simulink model "Even_Software_rezontor_original"  (R2019a)
settings: Solver=VariableStepAuto  StartTime=0.0  StopTime=20  FixedStep=0.000001  RelTol=1e-3
libraries: simulink x1
settings Model: NumberOfSteps=16  Creator=vardhah  LastModifiedBy=vardhah
settings DataIOCC: ReturnWorkspaceOutputs=off
settings DebuggingCC: UnderSpecifiedDimensionMsg=warning  ArithmeticOperatorsInVariantConditions=warning

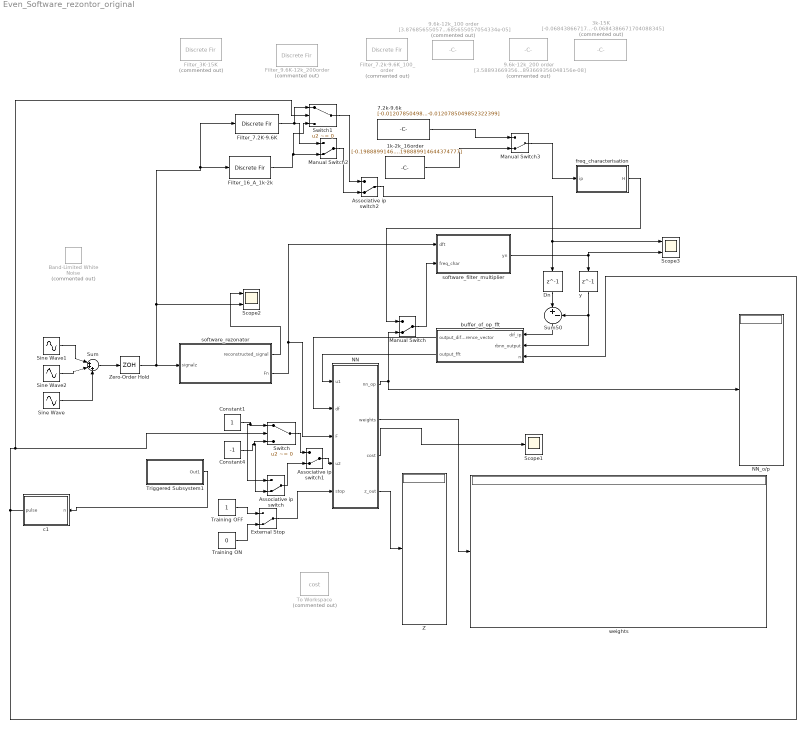
== system Even_Software_rezontor_original ==
  1k-2k_16order : Constant  Value=[-0.198889914644374777 0.0882189428518377339 0.0736891495871065116 0.0638368801789635787 0.0566372642221577294 0.0523172683654103132 0.0494565343907736044 0.048157521822162791 0.048157521822162791 0.0494565343907736044 0.0523172683654103132 0.0566372642221577294 0.0638368801789635787 0.0736891495871065116 0.0882189428518377339 -0.198889914644374777]  VectorParams1D=off
  3k-15K : Constant  Commented=on  Value=[-0.0684386671704088345 -0.0216035519389094557 -0.0869907772510868094 -0.0695372998678755599 0.0160068430386171648 -0.171506412844009415 -0.104404398490726372 0.48413102780480427 0.48413102780480427 -0.104404398490726372 -0.171506412844009415 0.0160068430386171648 -0.0695372998678755599 -0.0869907772510868094 -0.0216035519389094557 -0.0684386671704088345]  VectorParams1D=off
  "7.2k-9.6k " : Constant  Value=[-0.0120785049852322399 -0.0942455273574688279 0.0101245004695954266 0.125460404555770566 0.034165372769331126 -0.1614987160724079 -0.0984930555982914957 0.150982315564688691 0.150982315564688691 -0.0984930555982914957 -0.1614987160724079 0.034165372769331126 0.125460404555770566 0.0101245004695954266 -0.0942455273574688279 -0.0120785049852322399]  VectorParams1D=off
  9.6k-12k_100 order : Constant  Commented=on  Value=[3.87685655057054334e-05 0.000108803053226908729 -8.26167990877867136e-05 -0.000293336203733274498 2.6285942662608911e-05 0.000470643257144739719 0.000128704829547001234 -0.000409932472117148169 -0.000168878837800233775 5.29388077798551043e-06 -0.000285438581748162664 0.000476496961661710902 0.00138356120682394616 -0.000476433595901257331 -0.00260989841330203781 -0.000263832520003181659 0.00288776740876196033 0.00103696232298899297 -0.00148535664212565491 -0.00029781571721707251 -0.000910294888597508478 -0.00301220003423313329 0.00221471961553778218 0.00782175074594450466 -0.000709211369068674449 -0.0107696105008747954 -0.00258145844866515843 0.00855726436285330835 0.00338081517511367325 -0.00144715698429817813 0.00287506321799563301 -0.00544178445149644165 -0.016125692798747971 0.00552050119563736973 0.0291833518348223603 0.00265487109805798843 -0.0313375380418604021 -0.0109425432817974923 0.0170337904278449956 0.00463136074451602191 0.00673385154025073988 0.0271658069884841494 -0.0215094126752095813 -0.080672987166974186 0.00848125715451410883 0.135328268501058141 0.0372155688614851238 -0.164113227506699488 -0.099857601639362345 0.150463696417151488 0.150463696417151488 -0.099857601639362345 -0.164113227506699488 0.0372155688614851238 0.135328268501058141 0.00848125715451410883 -0.080672987166974186 -0.0215094126752095813 0.0271658069884841494 0.00673385154025073988 0.00463136074451602191 0.0170337904278449956 -0.0109425432817974923 -0.0313375380418604021 0.00265487109805798843 0.0291833518348223603 0.00552050119563736973 -0.016125692798747971 -0.00544178445149644165 0.00287506321799563301 -0.00144715698429817813 0.00338081517511367325 0.00855726436285330835 -0.00258145844866515843 -0.0107696105008747954 -0.000709211369068674449 0.00782175074594450466 0.00221471961553778218 -0.00301220003423313329 -0.000910294888597508478 -0.00029781571721707251 -0.00148535664212565491 0.00103696232298899297 0.00288776740876196033 -0.000263832520003181659 -0.00260989841330203781 -0.000476433595901257331 0.00138356120682394616 0.000476496961661710902 -0.000285438581748162664 5.29388077798551043e-06 -0.000168878837800233775 -0.000409932472117148169 0.000128704829547001234 0.000470643257144739719 2.6285942662608911e-05 -0.000293336203733274498 -8.26167990877867136e-05 0.000108803053226908729 3.87685655057054334e-05]  VectorParams1D=off
  9.6k-12k_200 order : Constant  Commented=on  Value=[3.58893669356048156e-08 -3.82818873463390521e-08 -2.0321720028023873e-07 4.90359188072874186e-08 5.60695246712035587e-07 1.09660540028249228e-07 -9.02554244437910404e-07 -4.11425973326973434e-07 7.02261176603049468e-07 1.84471216608655933e-07 3.26725285155721724e-07 1.85122942566739851e-06 -1.30883758906231066e-06 -6.26130099657902526e-06 3.05461039932901012e-07 1.09009807667638867e-05 3.23497432520277999e-06 -1.08958455239369133e-05 -4.97738604970975483e-06 2.96863479339988865e-06 -4.0832027868080837e-06 8.18297554751245384e-06 2.96530358064679952e-05 -9.55109847507026519e-06 -6.23922165547140565e-05 -7.71216677200245448e-06 7.59750359409520817e-05 2.93209615001356784e-05 -4.65187720652641962e-05 -1.41370609590419019e-05 -1.56985235131491563e-05 -7.53719240448361523e-05 5.59153495137252289e-05 0.000221327384655395267 -1.66050969068338295e-05 -0.000328656395451828759 -8.51260959631819787e-05 0.000282645117406031716 0.000119666235755805559 -6.72511324233616883e-05 7.71213722411986897e-05 -0.000163098688300092245 -0.000529184616157781082 0.000174782969900715956 0.000998932721197958676 0.000103789032707165716 -0.00109406787912954759 -0.000393069844497760581 0.000605548903230077127 0.00017901057135702881 0.000188671213168486616 0.0008317537932211581 -0.000616428076574026661 -0.00225801358273229787 0.000189644939633113819 0.00309786671618311488 0.000749066198738662951 -0.00246959577998202753 -0.000999305917144800888 0.000543345759446133242 -0.000591058888909330575 0.00125474640273121702 0.00385350017895572799 -0.0012819719093164299 -0.00685815514325687284 -0.000643891365732486565 0.00710257598433050412 0.00245016739238454462 -0.00372825461824609263 -0.00107354982596571057 -0.00112558364252808812 -0.00473944354418633605 0.00351472715485449472 0.0123820578712038748 -0.0011101460878915094 -0.0164148510072775998 -0.00382732465676402251 0.0127139357915301426 0.00503981617377440537 -0.00272012803122949386 0.00293385456875478335 -0.00629326791759583608 -0.0189964846306969505 0.00647240842885716226 0.0339172426787937645 0.00302977722420997957 -0.0357411919442247455 -0.0123754194694439944 0.0194465496197908511 0.00571238915438039823 0.00633940801538525594 0.0275121602229752085 -0.0219528139243238031 -0.0822938722183100269 0.00864574898877375209 0.1372509242650502 0.0376134106872798024 -0.165584050427181245 -0.100574100965544921 0.151437569678198519 0.151437569678198519 -0.100574100965544921 -0.165584050427181245 0.0376134106872798024 0.1372509242650502 0.00864574898877375209 -0.0822938722183100269 -0.0219528139243238031 0.0275121602229752085 0.00633940801538525594 0.00571238915438039823 0.0194465496197908511 -0.0123754194694439944 -0.0357411919442247455 0.00302977722420997957 0.0339172426787937645 0.00647240842885716226 -0.0189964846306969505 -0.00629326791759583608 0.00293385456875478335 -0.00272012803122949386 0.00503981617377440537 0.0127139357915301426 -0.00382732465676402251 -0.0164148510072775998 -0.0011101460878915094 0.0123820578712038748 0.00351472715485449472 -0.00473944354418633605 -0.00112558364252808812 -0.00107354982596571057 -0.00372825461824609263 0.00245016739238454462 0.00710257598433050412 -0.000643891365732486565 -0.00685815514325687284 -0.0012819719093164299 0.00385350017895572799 0.00125474640273121702 -0.000591058888909330575 0.000543345759446133242 -0.000999305917144800888 -0.00246959577998202753 0.000749066198738662951 0.00309786671618311488 0.000189644939633113819 -0.00225801358273229787 -0.000616428076574026661 0.0008317537932211581 0.000188671213168486616 0.00017901057135702881 0.000605548903230077127 -0.000393069844497760581 -0.00109406787912954759 0.000103789032707165716 0.000998932721197958676 0.000174782969900715956 -0.000529184616157781082 -0.000163098688300092245 7.71213722411986897e-05 -6.72511324233616883e-05 0.000119666235755805559 0.000282645117406031716 -8.51260959631819787e-05 -0.000328656395451828759 -1.66050969068338295e-05 0.000221327384655395267 5.59153495137252289e-05 -7.53719240448361523e-05 ...(+757 chars)]  VectorParams1D=off
  Associative ip switch : ManualSwitch  CurrentSetting=0
  Associative ip switch1 : ManualSwitch  CurrentSetting=0
  Associative ip switch2 : ManualSwitch  CurrentSetting=0
  Band-Limited White Noise : simulink/Sources/Band-Limited White Noise  Commented=on  Cov=[2]  Ts=0.000001  seed=[23341]
  Constant1 : Constant
  Constant4 : Constant  Value=-1
  Dn : Delay  DelayLength=1  InitialCondition=0
  External Stop : ManualSwitch  CurrentSetting=0
  Filter_16_A_1k-2k : DiscreteFir  Tag=BlockMethodSubSystem  Coefficients=[-0.198889914644374777 0.0882189428518377339 0.0736891495871065116 0.0638368801789635787 0.0566372642221577294 0.0523172683654103132 0.0494565343907736044 0.048157521822162791 0.048157521822162791 0.0494565343907736044 0.0523172683654103132 0.0566372642221577294 0.0638368801789635787 0.0736891495871065116 0.0882189428518377339 -0.198889914644374777]  InputProcessing=Columns as channels (frame based)
  Filter_3K-15K : DiscreteFir  Tag=BlockMethodSubSystem  Commented=on  Coefficients=[-0.0684386671704088345 -0.0216035519389094557 -0.0869907772510868094 -0.0695372998678755599 0.0160068430386171648 -0.171506412844009415 -0.104404398490726372 0.48413102780480427 0.48413102780480427 -0.104404398490726372 -0.171506412844009415 0.0160068430386171648 -0.0695372998678755599 -0.0869907772510868094 -0.0216035519389094557 -0.0684386671704088345]  InputProcessing=Columns as channels (frame based)
  "Filter_7.2K-9.6K " : DiscreteFir  Tag=BlockMethodSubSystem  Coefficients=[-0.0120785049852322399 -0.0942455273574688279 0.0101245004695954266 0.125460404555770566 0.034165372769331126 -0.1614987160724079 -0.0984930555982914957 0.150982315564688691 0.150982315564688691 -0.0984930555982914957 -0.1614987160724079 0.034165372769331126 0.125460404555770566 0.0101245004695954266 -0.0942455273574688279 -0.0120785049852322399]  InputProcessing=Columns as channels (frame based)
  Filter_7.2k-9.6K_100_order : DiscreteFir  Tag=BlockMethodSubSystem  Commented=on  Coefficients=[3.87685655057054334e-05 0.000108803053226908729 -8.26167990877867136e-05 -0.000293336203733274498 2.6285942662608911e-05 0.000470643257144739719 0.000128704829547001234 -0.000409932472117148169 -0.000168878837800233775 5.29388077798551043e-06 -0.000285438581748162664 0.000476496961661710902 0.00138356120682394616 -0.000476433595901257331 -0.00260989841330203781 -0.000263832520003181659 0.00288776740876196033 0.00103696232298899297 -0.00148535664212565491 -0.00029781571721707251 -0.000910294888597508478 -0.00301220003423313329 0.00221471961553778218 0.00782175074594450466 -0.000709211369068674449 -0.0107696105008747954 -0.00258145844866515843 0.00855726436285330835 0.00338081517511367325 -0.00144715698429817813 0.00287506321799563301 -0.00544178445149644165 -0.016125692798747971 0.00552050119563736973 0.0291833518348223603 0.00265487109805798843 -0.0313375380418604021 -0.0109425432817974923 0.0170337904278449956 0.00463136074451602191 0.00673385154025073988 0.0271658069884841494 -0.0215094126752095813 -0.080672987166974186 0.00848125715451410883 0.135328268501058141 0.0372155688614851238 -0.164113227506699488 -0.099857601639362345 0.150463696417151488 0.150463696417151488 -0.099857601639362345 -0.164113227506699488 0.0372155688614851238 0.135328268501058141 0.00848125715451410883 -0.080672987166974186 -0.0215094126752095813 0.0271658069884841494 0.00673385154025073988 0.00463136074451602191 0.0170337904278449956 -0.0109425432817974923 -0.0313375380418604021 0.00265487109805798843 0.0291833518348223603 0.00552050119563736973 -0.016125692798747971 -0.00544178445149644165 0.00287506321799563301 -0.00144715698429817813 0.00338081517511367325 0.00855726436285330835 -0.00258145844866515843 -0.0107696105008747954 -0.000709211369068674449 0.00782175074594450466 0.00221471961553778218 -0.00301220003423313329 -0.000910294888597508478 -0.00029781571721707251 -0.00148535664212565491 0.00103696232298899297 0.00288776740876196033 -0.000263832520003181659 -0.00260989841330203781 -0.000476433595901257331 0.00138356120682394616 0.000476496961661710902 -0.000285438581748162664 5.29388077798551043e-06 -0.000168878837800233775 -0.000409932472117148169 0.000128704829547001234 0.000470643257144739719 2.6285942662608911e-05 -0.000293336203733274498 -8.26167990877867136e-05 0.000108803053226908729 3.87685655057054334e-05]  InputProcessing=Columns as channels (frame based)
  Filter_9.6K-12k_200order : DiscreteFir  Tag=BlockMethodSubSystem  Commented=on  Coefficients=[3.58893669356048156e-08 -3.82818873463390521e-08 -2.0321720028023873e-07 4.90359188072874186e-08 5.60695246712035587e-07 1.09660540028249228e-07 -9.02554244437910404e-07 -4.11425973326973434e-07 7.02261176603049468e-07 1.84471216608655933e-07 3.26725285155721724e-07 1.85122942566739851e-06 -1.30883758906231066e-06 -6.26130099657902526e-06 3.05461039932901012e-07 1.09009807667638867e-05 3.23497432520277999e-06 -1.08958455239369133e-05 -4.97738604970975483e-06 2.96863479339988865e-06 -4.0832027868080837e-06 8.18297554751245384e-06 2.96530358064679952e-05 -9.55109847507026519e-06 -6.23922165547140565e-05 -7.71216677200245448e-06 7.59750359409520817e-05 2.93209615001356784e-05 -4.65187720652641962e-05 -1.41370609590419019e-05 -1.56985235131491563e-05 -7.53719240448361523e-05 5.59153495137252289e-05 0.000221327384655395267 -1.66050969068338295e-05 -0.000328656395451828759 -8.51260959631819787e-05 0.000282645117406031716 0.000119666235755805559 -6.72511324233616883e-05 7.71213722411986897e-05 -0.000163098688300092245 -0.000529184616157781082 0.000174782969900715956 0.000998932721197958676 0.000103789032707165716 -0.00109406787912954759 -0.000393069844497760581 0.000605548903230077127 0.00017901057135702881 0.000188671213168486616 0.0008317537932211581 -0.000616428076574026661 -0.00225801358273229787 0.000189644939633113819 0.00309786671618311488 0.000749066198738662951 -0.00246959577998202753 -0.000999305917144800888 0.000543345759446133242 -0.000591058888909330575 0.00125474640273121702 0.00385350017895572799 -0.0012819719093164299 -0.00685815514325687284 -0.000643891365732486565 0.00710257598433050412 0.00245016739238454462 -0.00372825461824609263 -0.00107354982596571057 -0.00112558364252808812 -0.00473944354418633605 0.00351472715485449472 0.0123820578712038748 -0.0011101460878915094 -0.0164148510072775998 -0.00382732465676402251 0.0127139357915301426 0.00503981617377440537 -0.00272012803122949386 0.00293385456875478335 -0.00629326791759583608 -0.0189964846306969505 0.00647240842885716226 0.0339172426787937645 0.00302977722420997957 -0.0357411919442247455 -0.0123754194694439944 0.0194465496197908511 0.00571238915438039823 0.00633940801538525594 0.0275121602229752085 -0.0219528139243238031 -0.0822938722183100269 0.00864574898877375209 0.1372509242650502 0.0376134106872798024 -0.165584050427181245 -0.100574100965544921 0.151437569678198519 0.151437569678198519 -0.100574100965544921 -0.165584050427181245 0.0376134106872798024 0.1372509242650502 0.00864574898877375209 -0.0822938722183100269 -0.0219528139243238031 0.0275121602229752085 0.00633940801538525594 0.00571238915438039823 0.0194465496197908511 -0.0123754194694439944 -0.0357411919442247455 0.00302977722420997957 0.0339172426787937645 0.00647240842885716226 -0.0189964846306969505 -0.00629326791759583608 0.00293385456875478335 -0.00272012803122949386 0.00503981617377440537 0.0127139357915301426 -0.00382732465676402251 -0.0164148510072775998 -0.0011101460878915094 0.0123820578712038748 0.00351472715485449472 -0.00473944354418633605 -0.00112558364252808812 -0.00107354982596571057 -0.00372825461824609263 0.00245016739238454462 0.00710257598433050412 -0.000643891365732486565 -0.00685815514325687284 -0.0012819719093164299 0.00385350017895572799 0.00125474640273121702 -0.000591058888909330575 0.000543345759446133242 -0.000999305917144800888 -0.00246959577998202753 0.000749066198738662951 0.00309786671618311488 0.000189644939633113819 -0.00225801358273229787 -0.000616428076574026661 0.0008317537932211581 0.000188671213168486616 0.00017901057135702881 0.000605548903230077127 -0.000393069844497760581 -0.00109406787912954759 0.000103789032707165716 0.000998932721197958676 0.000174782969900715956 -0.000529184616157781082 -0.000163098688300092245 7.71213722411986897e-05 -6.72511324233616883e-05 0.000119666235755805559 0.000282645117406031716 -8.51260959631819787e-05 -0.000328656395451828759 -1.66050969068338295e-05 0.000221327384655395267 5.59153495137252289e-05 -7.53719240448361523e-05 ...(+757 chars)]  InputProcessing=Columns as channels (frame based)
  Manual Switch : ManualSwitch  CurrentSetting=0  varsize=on
  Manual Switch2 : ManualSwitch  CurrentSetting=0
  Manual Switch3 : ManualSwitch  CurrentSetting=0
  NN : MATLAB Function  TreatAsAtomicUnit=on
  NN_o/p : Display
  Scope1 : Scope
  Scope2 : Scope  NumInputPorts=2
  Scope3 : Scope  NumInputPorts=2
  Sine Wave : Sin  Amplitude=3  Frequency=50  SampleTime=0
  Sine Wave1 : Sin  Amplitude=3  Frequency=200  SampleTime=0
  Sine Wave2 : Sin  Amplitude=3  Frequency=100  SampleTime=0
  Sum : Sum  Inputs=|+++
  Sum50 : Sum  Inputs=|+-
  Switch : Switch  Criteria=u2 ~= 0
  Switch1 : Switch  Criteria=u2 ~= 0
  To Workspace : ToWorkspace  Commented=on  VariableName=cost  SampleTime=-1
      settings: Save2DSignal=2-D array (concatenate along first dimension)
  Training OFF : Constant
  Training ON : Constant  Value=0
  Triggered Subsystem1 : Subsystem  TreatAsAtomicUnit=on
  Z : Display
  Zero-Order Hold : ZeroOrderHold  SampleTime=0.0001
  buffer_of_op_fft : MATLAB Function  TreatAsAtomicUnit=on
  c1 : MATLAB Function  TreatAsAtomicUnit=on
  freq_characterisation : MATLAB Function  TreatAsAtomicUnit=on
  software_filter_multiplier : MATLAB Function  TreatAsAtomicUnit=on
  software_rezonator : MATLAB Function  TreatAsAtomicUnit=on
  weights : Display
  y : Delay  DelayLength=1  InitialCondition=0
  wires:
  software_rezonator/1(reconstructed_signal) -> Scope2/1
  software_rezonator/2(Fn) -> software_filter_multiplier/1(dft), NN/3(F)
  software_filter_multiplier/1(yn) -> Scope3/2, y/1
  Zero-Order Hold/1 -> Scope2/2, "Filter_7.2K-9.6K "/1, Filter_16_A_1k-2k/1, software_rezonator/1(signalz)
  Sine Wave1/1 -> Sum/1
  Sine Wave2/1 -> Sum/2
  Sine Wave/1 -> Sum/3
  Sum/1 -> Zero-Order Hold/1
  Filter_16_A_1k-2k/1 -> Switch1/3, Manual Switch2/2
  Dn/1 -> Sum50/1
  y/1 -> buffer_of_op_fft/2(rbnn_output), Sum50/2
  Manual Switch/1 -> software_filter_multiplier/2(freq_char)
  freq_characterisation/1(H) -> Manual Switch/1
  NN/1(nn_op) -> Manual Switch/2, NN_o/p/1
  External Stop/1 -> NN/5(stop)
  Training OFF/1 -> External Stop/1
  Training ON/1 -> External Stop/2
  Constant4/1 -> Switch/3, Associative ip switch/2
  NN/3(cost) -> Scope1/1
  NN/2(weights) -> weights/1
  NN/4(z_out) -> Z/1
  1k-2k_16order/1 -> Manual Switch3/2
  "7.2k-9.6k "/1 -> Manual Switch3/1
  Manual Switch3/1 -> freq_characterisation/1(ip)
  Triggered Subsystem1/1(Out1) -> c1/1(n)
  c1/1(pulse) -> Switch/2, Switch1/2, buffer_of_op_fft/3(n)
  "Filter_7.2K-9.6K "/1 -> Switch1/1, Manual Switch2/1
  Switch/1 -> Associative ip switch1/1
  Associative ip switch1/1 -> NN/4(u2)
  Associative ip switch/1 -> Associative ip switch1/2
  Associative ip switch2/1 -> Scope3/1, Dn/1
  Switch1/1 -> Associative ip switch2/1
  Manual Switch2/1 -> Associative ip switch2/2
  Constant1/1 -> Switch/1, Associative ip switch/1
  Sum50/1 -> buffer_of_op_fft/1(dif_ip)
  buffer_of_op_fft/1(output_difference_vector) -> NN/2(df)
  buffer_of_op_fft/2(output_fft) -> NN/1(u1)

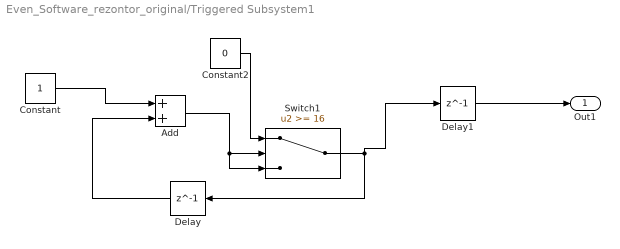
== system Even_Software_rezontor_original/Triggered Subsystem1 ==
  Add : Sum
  Constant : Constant
  Constant2 : Constant  Value=0
  Delay : Delay  DelayLength=1  InitialCondition=0
  Delay1 : Delay  DelayLength=1  InitialCondition=0
  Switch1 : Switch  Threshold=16
  Out1 : Outport
  wires:
  Constant2/1 -> Switch1/1
  Constant/1 -> Add/1
  Switch1/1 -> Delay1/1, Delay/1
  Delay/1 -> Add/2
  Add/1 -> Switch1/3, Switch1/2
  Delay1/1 -> Out1/1

== matlab function Even_Software_rezontor_original/NN ==
  settings: sampleTime=0.01
  data: u1 input; df input; F input; u2 input; nn_op output; weights output; cost output; z_out output; stop input
function [nn_op,weights,cost,z_out]  = NN(u1,df,F,u2,stop)

persistent w1;
persistent vy;
persistent g;
persistent itr;
persistent J;
persistent del_w;
persistent mult;
persistent memory_alloc_flag;
persistent n;

alpha = 0.03;



%layer declaration
input_layer = 17; 
layer_1=16;


if isempty(w1)
       w1=randn(input_layer,layer_1)*0.2;
end

if isempty(n)
        n = 0; 
end
n=n+1;
if isempty(memory_alloc_flag)
        memory_alloc_flag = 0; 
end
if isempty(mult)
       mult=zeros(layer_1,layer_1*input_layer); 
end
if memory_alloc_flag==0
 %write memory allocation for looped code here.. 
 mult=[];
  for itr =1:layer_1
   mult=[mult;[zeros(1,(itr-1)*input_layer) ones(1,input_layer) zeros(1,(input_layer-itr-1)*input_layer)]];
 end
 memory_alloc_flag=1;
end

if isempty(del_w)
    del_w=zeros(1,272);
end

if isempty(itr)
    itr=0;
end
if isempty(J)
    J=0;
end

%gradient initialisation
if isempty(g)
    g= zeros(16,272);
   %g= rand(16,272);   
end


%prestored Vy matrix
if isempty(vy)
    vy=[0.0625000000000000,0.0625000000000000,0.0625000000000000,0.0625000000000000,0.0625000000000000,0.0625000000000000,0.0625000000000000,0.0625000000000000,0.0625000000000000,0.0625000000000000,0.0625000000000000,0.0625000000000000,0.0625000000000000,0.0625000000000000,0.0625000000000000,0.0625000000000000;0.0577424707819554,0.0441941738241592,0.0239177145228181,-1.14810637420064e-17,-0.0239177145228181,-0.0441941738241592,-0.0577424707819554,-0.0625000000000000,-0.0577424707819554,-0.0441941738241592,-0.0239177145228181,3.82702124733548e-18,0.0239177145228181,0.0441941738241592,0.0577424707819554,0.0625000000000000;0.0441941738241592,-2.67891487313484e-17,-0.0441941738241592,-0.0625000000000000,-0.0441941738241592,1.91351062366774e-17,0.0441941738241592,0.0625000000000000,0.0441941738241592,-1.14810637420064e-17,-0.0441941738241592,-0.0625000000000000,-0.0441941738241592,3.82702124733548e-18,0.0441941738241592,0.0625000000000000;0.0239177145228179,-0.0441941738241592,-0.0577424707819554,3.44431912260193e-17,0.0577424707819555,0.0441941738241592,-0.0239177145228182,-0.0625000000000000,-0.0239177145228181,0.0441941738241592,0.0577424707819554,-1.14810637420064e-17,-0.0577424707819554,-0.0441941738241592,0.0239177145228181,0.0625000000000000;-1.68427621172548e-16,-0.0625000000000000,-6.12710262471544e-17,0.0625000000000000,-1.53119536183206e-16,-0.0625000000000000,3.44431912260193e-17,0.0625000000000000,-2.67891487313484e-17,-0.0625000000000000,1.91351062366774e-17,0.0625000000000000,-1.14810637420064e-17,-0.0625000000000000,3.82702124733548e-18,0.0625000000000000;-0.0239177145228182,-0.0441941738241591,0.0577424707819554,-1.68427621172548e-16,-0.0577424707819554,0.0441941738241592,0.0239177145228181,-0.0625000000000000,0.0239177145228182,0.0441941738241592,-0.0577424707819554,1.91351062366774e-17,0.0577424707819554,-0.0441941738241592,-0.0239177145228181,0.0625000000000000;-0.0441941738241596,-3.06548562684706e-17,0.0441941738241593,-0.0625000000000000,0.0441941738241594,-1.68427621172548e-16,-0.0441941738241592,0.0625000000000000,-0.0441941738241592,3.44431912260193e-17,0.0441941738241592,-0.0625000000000000,0.0441941738241592,-1.14810637420064e-17,-0.0441941738241592,0.0625000000000000;-0.0577424707819556,0.0441941738241594,-0.0239177145228178,-3.06548562684706e-17,0.0239177145228179,-0.0441941738241591,0.0577424707819554,-0.0625000000000000,0.0577424707819555,-0.0441941738241592,0.0239177145228182,-2.67891487313484e-17,-0.0239177145228181,0.0441941738241592,-0.0577424707819554,0.0625000000000000;-0.0625000000000000,0.0625000000000000,-0.0625000000000000,0.0625000000000000,-0.0625000000000000,0.0625000000000000,-0.0625000000000000,0.0625000000000000,-0.0625000000000000,0.0625000000000000,-0.0625000000000000,0.0625000000000000,-0.0625000000000000,0.0625000000000000,-0.0625000000000000,0.0625000000000000;-0.0239177145228184,0.0441941738241592,-0.0577424707819555,0.0625000000000000,-0.0577424707819553,0.0441941738241592,-0.0239177145228180,-6.88863824520386e-17,0.0239177145228181,-0.0441941738241593,0.0577424707819554,-0.0625000000000000,0.0577424707819554,-0.0441941738241592,0.0239177145228181,0;-0.0441941738241594,0.0625000000000000,-0.0441941738241593,-3.36855242345096e-16,0.0441941738241595,-0.0625000000000000,0.0441941738241592,7.65404249467096e-17,-0.0441941738241593,0.0625000000000000,-0.0441941738241592,-3.82702124733548e-17,0.0441941738241593,-0.0625000000000000,0.0441941738241592,0;-0.0577424707819556,0.0441941738241592,0.0239177145228178,-0.0625000000000000,0.0239177145228177,0.0441941738241592,-0.0577424707819555,-3.06239072366412e-16,0.0577424707819554,-0.0441941738241592,-0.0239177145228181,0.0625000000000000,-0.0239177145228181,-0.0441941738241593,0.0577424707819554,0;-0.0625000000000000,6.13097125369412e-17,0.0625000000000000,1.37772764904077e-16,-0.0625000000000000,-3.36855242345096e-16,0.0625000000000000,9.18485099360515e-17,-0.0625000000000000,-6.88863824520386e-17,0.0625000000000000,4.59242549680257e-17,-0.0625000000000000,-2.29621274840129e-17,0.0625000000000000,0;-0.0577424707819553,-0.0441941738241594,0.0239177145228181,0.0625000000000000,0.0239177145228186,-0.0441941738241590,-0.0577424707819555,1.22542052494309e-16,0.0577424707819554,0.0441941738241593,-0.0239177145228180,-0.0625000000000000,-0.0239177145228182,0.0441941738241592,0.0577424707819554,0;-0.0441941738241587,-0.0625000000000000,-0.0441941738241588,6.13097125369412e-17,0.0441941738241588,0.0625000000000000,0.0441941738241592,1.07156594925393e-16,-0.0441941738241590,-0.0625000000000000,-0.0441941738241593,-5.35782974626967e-17,0.0441941738241592,0.0625000000000000,0.0441941738241592,0;-0.0239177145228178,-0.0441941738241593,-0.0577424707819556,-0.0625000000000000,-0.0577424707819556,-0.0441941738241594,-0.0239177145228184,-3.36855242345096e-16,0.0239177145228181,0.0441941738241592,0.0577424707819554,0.0625000000000000,0.0577424707819554,0.0441941738241593,0.0239177145228182,0;0,0,0,0,0,0,0,0,0,0,0,0,0,0,0,0];
end



%input initialisation
x_in = [real(u1(1)) real(u1(2)) real(u1(3)) real(u1(4)) real(u1(5)) real(u1(6)) real(u1(7)) real(u1(8)) real(u1(9)) imag(u1(1)) imag(u1(2)) imag(u1(3)) imag(u1(4)) imag(u1(5)) imag(u1(6)) imag(u1(7))];

%parameter intialisation 
v=transpose([x_in u2]);


%F=transpose([real(X0) 2*(real(X1)*cos(pi*1*n/8)-imag(X1)*sin(pi*1*n/8)) 2*(real(X2)*cos(pi*2*n/8)-imag(X2)*sin(pi*2*n/8)) 2*(real(X3)*cos(pi*3*n/8)-imag(X3)*sin(pi*3*n/8)) 2*(real(X4)*cos(pi*4*n/8)-imag(X4)*sin(pi*4*n/8)) 2*(real(X5)*cos(pi*5*n/8)-imag(X5)*sin(pi*5*n/8)) 2*(real(X6)*cos(pi*6*n/8)-imag(X6)*sin(pi*6*n/8)) 2*(real(X7)*cos(pi*7*n/8)-imag(X7)*sin(pi*7*n/8)) -1^n*real(X8) -2*(imag(X9)*cos(pi*9*n/8)+real(X9)*sin(pi*9*n/8)) -2*(imag(X10)*cos(pi*10*n/8)+real(X10)*sin(pi*10*n/8)) -2*(imag(X11)*cos(pi*11*n/8)+real(X11)*sin(pi*11*n/8)) -2*(imag(X12)*cos(pi*12*n/8)+real(X12)*sin(pi*12*n/8)) -2*(imag(X13)*cos(pi*13*n/8)+real(X13)*sin(pi*13*n/8)) -2*(imag(X14)*cos(pi*14*n/8)+real(X14)*sin(pi*14*n/8)) -2*(imag(X15)*cos(pi*15*n/8)+real(X15)*sin(pi*15*n/8))]); 
%u_out=v;


%forward propogation
z=w1'*v ;
z_out=z;
a=(1./(1+exp(-z)));
an=(a-0.5);

%calculation of Nv:
dz_a=a.*(1-a);                  
Nv=w1'.* repmat(dz_a,1, size(w1,1));

%calculation of aD
aD=transpose(F)*Nv*vy;
A=[aD;eye(15) zeros(15,1)];
B=[transpose(F) ; zeros(15,16)];   
dw1=v*transpose(dz_a);

%added to vectorise the implementation
Expanded_dw1=repmat(transpose(dw1),1,size(dw1,2));
Nw=Expanded_dw1.*mult; 
g=A*g+B*Nw;



if mod(n,16)==0 && stop==0
    del_w =alpha*df*1*g/16 ;
    del_w_reshaped= reshape(del_w,[17,16]);
    w1=w1+ del_w_reshaped;
    itr=itr+1;
    J= 1/32*sum(df.^2,'all');
end
cost=J;
weights=w1;


nn_op=an;


end

== matlab function Even_Software_rezontor_original/buffer_of_op_fft ==
  data: output_difference_vector output size=[1,16]; output_fft output size=[1,16]; dif_ip input; rbnn_output input; n input
function [output_difference_vector,output_fft] = difBuffer(dif_ip,rbnn_output,n)                      

 sz=16;                       % size of the dft 
 
 persistent a;
 persistent b;
 if isempty(b)
  b= zeros(1,sz);
 end
 if isempty(a)
  a= zeros(1,sz);
 end
if n==1 
  a=zeros(1,sz);
  b= zeros(1,sz);
 else
  a= circshift(a,1);
  a(1)=dif_ip;
  b= circshift(b,1);
  b(1)=rbnn_output;
 end
 output_difference_vector=a; 
 output_fft=1/sz*fft(b); 
end

== matlab function Even_Software_rezontor_original/freq_characterisation ==
  data: ip input; H output
function H  = freq_character(ip)                      

dft_of_ip=fft(ip); 
size_dft=size(dft_of_ip,2)/2;
H =transpose([real(dft_of_ip(1:size_dft+1)) imag(dft_of_ip(2:size_dft))]);

end

== matlab function Even_Software_rezontor_original/software_rezonator ==
  data: signalz input; reconstructed_signal output; Fn output size=16
function [reconstructed_signal,Fn]   = rezonator(signalz)

persistent numberofrezonator;
persistent g c bfr_rezo_sm aft_delay dft_out;
persistent out signal_dif;
persistent n;
persistent memory_alloc_flag;


%assign the number of rezonator here. For configuring it for higher order
%rezonator  we need to change (1) 'numberofrezonaotor' variable
if isempty(numberofrezonator)
        numberofrezonator = 16;   %here 16 parallel rezonators
end

%Initialisation of memory allocations/variables ====> 
if isempty(memory_alloc_flag)
        memory_alloc_flag = 0; 
end
if isempty(g)
       g=zeros(numberofrezonator,numberofrezonator,'like',0i); 
end
if isempty(c)
       c=zeros(numberofrezonator,numberofrezonator,'like',0i); 
end
if memory_alloc_flag==0
 for i=0:numberofrezonator-1
  for j= 0:numberofrezonator-1
   g(i+1,j+1)=1/numberofrezonator*(exp(-1i*2*pi*i*j/numberofrezonator));
   c(i+1,j+1)=(exp(1i*2*pi*i*j/numberofrezonator));
  end 
 end
 memory_alloc_flag=1;
end


%Initialisation of variables  =====> 
if isempty(n)
        n = 0;   
end 
if isempty(out)
  out=0+0i;
end
if isempty(signal_dif)
  signal_dif=0+0i;
end
if isempty(bfr_rezo_sm)
  bfr_rezo_sm=repmat(0+0i,numberofrezonator,1);
end
if isempty(aft_delay)
  aft_delay=repmat(0+0i,numberofrezonator,1);
end
if isempty(dft_out)
  dft_out=repmat(0+0i,numberofrezonator,1);
end

%creating cycle of rotation for selection of correct column of g & c.
cycle=mod(n,numberofrezonator);

%resonator core -----------------------------> 
dft_out=c(:,cycle+1).*aft_delay;
out= sum(dft_out,1);
signal_dif=signalz-out;
bfr_rezo_sm=g(:,cycle+1).*signal_dif;

%counting the counter
n=n+1;

% output assignment ------------------>
reconstructed_signal=out;
dft=aft_delay; 
N=size(dft,1);
a=1:1:N/2-1;
b=N/2+1:1:N-1;
dft_trans=transpose(dft);
Fn=transpose([real(dft_trans(1)) 2*(real(dft_trans(2:N/2)).*cos(2*pi*a*n/N)-imag(dft_trans(2:N/2)).*sin(2*pi*a*n/N)) -1^n*real(dft_trans(N/2+1)) -2*(imag(dft_trans(N/2+2:N)).*cos(2*pi*b*n/N)+real(dft_trans(N/2+2:N)).*sin(2*pi*b*n/N))]);
%--------output assignment over----------<

%final updation of buffer ------>>>>>>>>>>>>
aft_delay= aft_delay+bfr_rezo_sm; 
end

== matlab function Even_Software_rezontor_original/software_filter_multiplier ==
  data: dft input; yn output; freq_char input
function yn = fcn(dft,freq_char)
yn=transpose(freq_char)*dft;
end

== matlab function Even_Software_rezontor_original/c1 ==
  data: n input; pulse output
function pulse  = fcn(n)
persistent cnt counter;
if isempty(cnt)
    cnt=0;
end
if isempty(counter)
    counter=0;
end


if n==15
     cnt=cnt+1;
end

 pulse = mod(cnt,2);
end
